simulink model "Model"  (R2024b)
settings: Solver=ode45  StartTime=0.0  StopTime=10.0  RelTol=1e-3
InitFcn:
  | Main
values from neighbouring files (symbols this model uses):
  A = [0, 1; 0, -20]    [Main.m]
  B = [0; 60]    [Main.m]
  C = [1, 0]    [Main.m]
  D = 0    [Main.m]
  K = K(4:5)    [Main.m]
  W0 = 6    [Main.m]
undefined symbols (not defined in the file or in its folder): H, RD
settings Model: Creator=Banaan  LastModifiedBy=Banaan

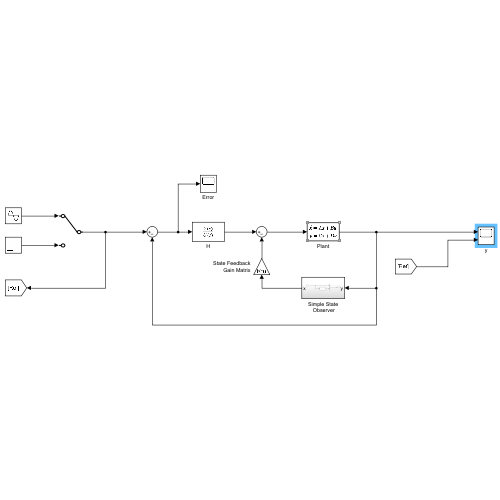
[thumbnail: Simulink's stored preview of the top-level diagram]
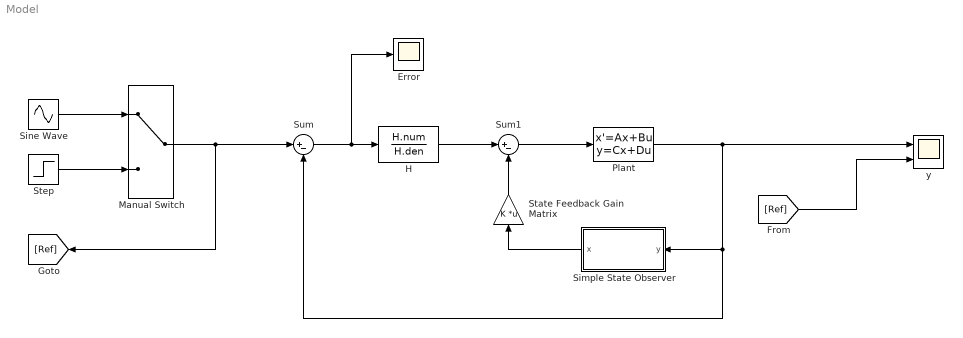
== system Model ==
  Error : Scope
  H : TransferFcn  Numerator=H.num  Denominator=H.den
  Manual Switch : ManualSwitch
  Plant : StateSpace  A=A  B=B  C=C  D=D  InitialCondition=0
  Simple State Observer : Subsystem
  Sine Wave : Sin  Frequency=W0  SampleTime=0
  State Feedback Gain Matrix : Gain  Gain=K  Multiplication=Matrix(K*u)
  Step : Step  After=50  SampleTime=0
  Sum : Sum  Inputs=|+-
  Sum1 : Sum  Inputs=|+-
  y : Scope  NumInputPorts=2
  wires:
  State Feedback Gain Matrix/1 -> Sum1/2
  Plant/1 -> y/1, Sum/2, Simple State Observer/1(y)
  Sum/1 -> H/1, Error/1
  Manual Switch/1 -> Sum/1, [Ref]
  Sum1/1 -> Plant/1
  H/1 -> Sum1/1
  Sine Wave/1 -> Manual Switch/1
  Step/1 -> Manual Switch/2
  Simple State Observer/1(x) -> State Feedback Gain Matrix/1
  [Ref] -> y/2

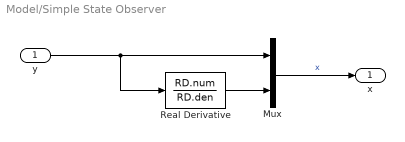
== system Model/Simple State Observer ==
  y : Inport
  Mux : Mux  Inputs=2
  Real Derivative : TransferFcn  Numerator=RD.num  Denominator=RD.den
  x : Outport
  wires:
  Real Derivative/1 -> Mux/2
  y/1 -> Real Derivative/1, Mux/1
  Mux/1 -> x/1  "x"
